simulink model "LGS_allFaultStuffDeleted"  (R2019b)
settings: Solver=FixedStepDiscrete  StartTime=0.0  StopTime=45.0  FixedStep=0.1  RelTol=1e-3
model workspace (MAT data in the model file):
  fipData : object (value not decoded)
  fipName : object (value not decoded)
  stepSize = 0.1
libraries: commrandsrc3 x16, simulink x3, LibFailureCondition x1
(part 5 of 7)

== stateflow chart LGS_allFaultStuffDeleted/Digital Part/Computing module1/GenericMonitoring8/GenericMonitoring2 ==
  state SensorValid
    entry: anomaly = false;
  state Channel1Invalid
  state SensorInvalid
    entry: anomaly = true;
  note: If at t the three channels are considered as valid and are equal, then the
      | value considered by the control software is this common value.
  state Channel2Invalid
  note: If a channel has been eliminated previously, and if at t the two remaining
      | channels are not equal, then the sensor is definitely considered as invalid.
  state Channel3Invalid
  note: If at t one channel is different from the two others for the first time (i.e.,
      | the three channels were considered as valid up to t), then this channel is
      | considered as invalid and is definitely eliminated. Only the two remaining
      | channels are considered in the future. At time t, the value considered by the
      | control software is the common value of the two remaining channels.
  (default) -> SensorValid
  SensorValid -> Channel1Invalid [order 1] : [(((Channel3&&Channel2) || ((~Channel3)&&(~Channel2))) && ((Channel1 && (~Channel2)) || ((~Channel1) && Channel2)))]
  Channel1Invalid -> SensorInvalid : [((Channel2 && (~Channel3)) || ((~Channel2) && Channel3))]
  SensorValid -> Channel2Invalid [order 2] : [(((Channel1&&Channel3) || ((~Channel1)&&(~Channel3))) && ((Channel1 && (~Channel2)) || ((~Channel1) && Channel2)))]
  SensorValid -> Channel3Invalid [order 3] : [(((Channel1&&Channel2) || ((~Channel1)&&(~Channel2))) && ((Channel1 && (~Channel3)) || ((~Channel1) && Channel3)))]
  Channel2Invalid -> SensorInvalid : [((Channel1 && (~Channel3)) || ((~Channel1) && Channel3))]
  Channel3Invalid -> SensorInvalid : [((Channel2 && (~Channel1)) || ((~Channel2) && Channel1))]
  data: Channel1 input boolean; Channel2 input boolean; Channel3 input boolean; anomaly output boolean

== stateflow chart LGS_allFaultStuffDeleted/Digital Part/Computing module1/GenericMonitoring9/GenericMonitoring2 ==
  state SensorValid
    entry: anomaly = false;
  state Channel1Invalid
  state SensorInvalid
    entry: anomaly = true;
  note: If at t the three channels are considered as valid and are equal, then the
      | value considered by the control software is this common value.
  state Channel2Invalid
  note: If a channel has been eliminated previously, and if at t the two remaining
      | channels are not equal, then the sensor is definitely considered as invalid.
  state Channel3Invalid
  note: If at t one channel is different from the two others for the first time (i.e.,
      | the three channels were considered as valid up to t), then this channel is
      | considered as invalid and is definitely eliminated. Only the two remaining
      | channels are considered in the future. At time t, the value considered by the
      | control software is the common value of the two remaining channels.
  (default) -> SensorValid
  SensorValid -> Channel1Invalid [order 1] : [(((Channel3&&Channel2) || ((~Channel3)&&(~Channel2))) && ((Channel1 && (~Channel2)) || ((~Channel1) && Channel2)))]
  Channel1Invalid -> SensorInvalid : [((Channel2 && (~Channel3)) || ((~Channel2) && Channel3))]
  SensorValid -> Channel2Invalid [order 2] : [(((Channel1&&Channel3) || ((~Channel1)&&(~Channel3))) && ((Channel1 && (~Channel2)) || ((~Channel1) && Channel2)))]
  SensorValid -> Channel3Invalid [order 3] : [(((Channel1&&Channel2) || ((~Channel1)&&(~Channel2))) && ((Channel1 && (~Channel3)) || ((~Channel1) && Channel3)))]
  Channel2Invalid -> SensorInvalid : [((Channel1 && (~Channel3)) || ((~Channel1) && Channel3))]
  Channel3Invalid -> SensorInvalid : [((Channel2 && (~Channel1)) || ((~Channel2) && Channel1))]
  data: Channel1 input boolean; Channel2 input boolean; Channel3 input boolean; anomaly output boolean

== stateflow chart LGS_allFaultStuffDeleted/Digital Part/Computing module1/GenericMonitoring15/GenericMonitoring2 ==
  state SensorValid
    entry: anomaly = false;
  state Channel1Invalid
  state SensorInvalid
    entry: anomaly = true;
  note: If at t the three channels are considered as valid and are equal, then the
      | value considered by the control software is this common value.
  state Channel2Invalid
  note: If a channel has been eliminated previously, and if at t the two remaining
      | channels are not equal, then the sensor is definitely considered as invalid.
  state Channel3Invalid
  note: If at t one channel is different from the two others for the first time (i.e.,
      | the three channels were considered as valid up to t), then this channel is
      | considered as invalid and is definitely eliminated. Only the two remaining
      | channels are considered in the future. At time t, the value considered by the
      | control software is the common value of the two remaining channels.
  (default) -> SensorValid
  SensorValid -> Channel1Invalid [order 1] : [(((Channel3&&Channel2) || ((~Channel3)&&(~Channel2))) && ((Channel1 && (~Channel2)) || ((~Channel1) && Channel2)))]
  Channel1Invalid -> SensorInvalid : [((Channel2 && (~Channel3)) || ((~Channel2) && Channel3))]
  SensorValid -> Channel2Invalid [order 2] : [(((Channel1&&Channel3) || ((~Channel1)&&(~Channel3))) && ((Channel1 && (~Channel2)) || ((~Channel1) && Channel2)))]
  SensorValid -> Channel3Invalid [order 3] : [(((Channel1&&Channel2) || ((~Channel1)&&(~Channel2))) && ((Channel1 && (~Channel3)) || ((~Channel1) && Channel3)))]
  Channel2Invalid -> SensorInvalid : [((Channel1 && (~Channel3)) || ((~Channel1) && Channel3))]
  Channel3Invalid -> SensorInvalid : [((Channel2 && (~Channel1)) || ((~Channel2) && Channel1))]
  data: Channel1 input boolean; Channel2 input boolean; Channel3 input boolean; anomaly output boolean

== stateflow chart LGS_allFaultStuffDeleted/Digital Part/Computing module1/GenericMonitoring16/GenericMonitoring2 ==
  state SensorValid
    entry: anomaly = false;
  state Channel1Invalid
  state SensorInvalid
    entry: anomaly = true;
  note: If at t the three channels are considered as valid and are equal, then the
      | value considered by the control software is this common value.
  state Channel2Invalid
  note: If a channel has been eliminated previously, and if at t the two remaining
      | channels are not equal, then the sensor is definitely considered as invalid.
  state Channel3Invalid
  note: If at t one channel is different from the two others for the first time (i.e.,
      | the three channels were considered as valid up to t), then this channel is
      | considered as invalid and is definitely eliminated. Only the two remaining
      | channels are considered in the future. At time t, the value considered by the
      | control software is the common value of the two remaining channels.
  (default) -> SensorValid
  SensorValid -> Channel1Invalid [order 1] : [(((Channel3&&Channel2) || ((~Channel3)&&(~Channel2))) && ((Channel1 && (~Channel2)) || ((~Channel1) && Channel2)))]
  Channel1Invalid -> SensorInvalid : [((Channel2 && (~Channel3)) || ((~Channel2) && Channel3))]
  SensorValid -> Channel2Invalid [order 2] : [(((Channel1&&Channel3) || ((~Channel1)&&(~Channel3))) && ((Channel1 && (~Channel2)) || ((~Channel1) && Channel2)))]
  SensorValid -> Channel3Invalid [order 3] : [(((Channel1&&Channel2) || ((~Channel1)&&(~Channel2))) && ((Channel1 && (~Channel3)) || ((~Channel1) && Channel3)))]
  Channel2Invalid -> SensorInvalid : [((Channel1 && (~Channel3)) || ((~Channel1) && Channel3))]
  Channel3Invalid -> SensorInvalid : [((Channel2 && (~Channel1)) || ((~Channel2) && Channel1))]
  data: Channel1 input boolean; Channel2 input boolean; Channel3 input boolean; anomaly output boolean

== stateflow chart LGS_allFaultStuffDeleted/Digital Part/Computing module2/AnalogicalSwitchMonitoring ==
  state SwitchOpened
    entry: time = int8(21);
    during: time = time -1;
  note: If the analogical switch is seen closed 1.5 second after a time interval of 20
      | seconds during which the handle position has not changed, then the switch
      | is considered as invalid.
  state Idle
    entry: anomaly = false;
  state HandleMoved
  state CounterOrder
  note: If the analogical switch is seen open 1 second after the handle position has
      | changed, then the switch is considered as invalid.
  state Anomaly
    entry: anomaly = true;
  (default) -> Idle
  SwitchOpened -> Idle [order 2] : [((time == 0) && (~SwitchSignal))]
  HandleMoved -> SwitchOpened [order 2] : [((SwitchSignal) && (~HandleMoved))]
  SwitchOpened -> CounterOrder [order 3] : [(HandleMoved)]
  SwitchOpened -> Anomaly [order 1] : [((time == 0) && (SwitchSignal))]
  Idle -> HandleMoved : [(HandleMoved)]
  HandleMoved -> CounterOrder [order 3] : [(HandleMoved)]
  CounterOrder -> HandleMoved
  HandleMoved -> Anomaly [order 1] : [((~SwitchSignal) && (~HandleMoved))]
  data: HandleMoved input boolean; time local int8 [0..21]; SwitchSignal input boolean; anomaly output boolean

== stateflow chart LGS_allFaultStuffDeleted/Digital Part/Computing module1/GenericMonitoring17/GenericMonitoring2 ==
  state SensorValid
    entry: anomaly = false;
  state Channel1Invalid
  state SensorInvalid
    entry: anomaly = true;
  note: If at t the three channels are considered as valid and are equal, then the
      | value considered by the control software is this common value.
  state Channel2Invalid
  note: If a channel has been eliminated previously, and if at t the two remaining
      | channels are not equal, then the sensor is definitely considered as invalid.
  state Channel3Invalid
  note: If at t one channel is different from the two others for the first time (i.e.,
      | the three channels were considered as valid up to t), then this channel is
      | considered as invalid and is definitely eliminated. Only the two remaining
      | channels are considered in the future. At time t, the value considered by the
      | control software is the common value of the two remaining channels.
  (default) -> SensorValid
  SensorValid -> Channel1Invalid [order 1] : [(((Channel3&&Channel2) || ((~Channel3)&&(~Channel2))) && ((Channel1 && (~Channel2)) || ((~Channel1) && Channel2)))]
  Channel1Invalid -> SensorInvalid : [((Channel2 && (~Channel3)) || ((~Channel2) && Channel3))]
  SensorValid -> Channel2Invalid [order 2] : [(((Channel1&&Channel3) || ((~Channel1)&&(~Channel3))) && ((Channel1 && (~Channel2)) || ((~Channel1) && Channel2)))]
  SensorValid -> Channel3Invalid [order 3] : [(((Channel1&&Channel2) || ((~Channel1)&&(~Channel2))) && ((Channel1 && (~Channel3)) || ((~Channel1) && Channel3)))]
  Channel2Invalid -> SensorInvalid : [((Channel1 && (~Channel3)) || ((~Channel1) && Channel3))]
  Channel3Invalid -> SensorInvalid : [((Channel2 && (~Channel1)) || ((~Channel2) && Channel1))]
  data: Channel1 input boolean; Channel2 input boolean; Channel3 input boolean; anomaly output boolean

== stateflow chart LGS_allFaultStuffDeleted/Digital Part/Computing module2/DoorMotionMonitoring ==
  state Idle
    entry: anomaly = false;
  state CloseDoors
    entry: time = int8(6);
    during: time = time -1;
  note: if the control software does not see the value door closed[x] = true for all
      | x ∈ {front, left, right} 7 seconds after stimulation of the closure electro-valve,
      | then the doors are considered as blocked and an anomaly is detected.
  state Succeeded
  state OpenDoors
    entry: time = int8(6);
    during: time = time - 1;
  note: if the control software does not see the value door open[x] = false for all x ∈ {front, left, right} 7 seconds after stimulation of the closure electro-valve, then the doors are considered as blocked and an anomaly is detected.
  state CounterOrder
  note: if the control software does not see the value door open[x] = true for all
      | x ∈ {front, left, right} 7 seconds after stimulation of the opening electrovalve,
      | then the doors are considered as blocked and an anomaly is detected.
  state DoorsBlocked
    entry: anomaly = true;
  note: if the control software does not see the value door closed[x] = false for all
      | x ∈ {front, left, right} 7 seconds after stimulation of the opening electro-valve,
      | then the doors are considered as blocked and an anomaly is detected.
  (default) -> Idle
  CloseDoors -> DoorsBlocked [order 2] : [((time == 0) && (~AllDoorsClosed))]
  Idle -> CloseDoors [order 2] : [((CloseDoorValve) && (~AllDoorsClosed))]
  CloseDoors -> DoorsBlocked [order 3] : [((time == 0) && (AllDoorsOpen))]
  Succeeded -> Idle
  CloseDoors -> Succeeded [order 1] : [(((time == 0) && (AllDoorsClosed)) && (~AllDoorsOpen))]
  CounterOrder -> CloseDoors [order 2] : [(CloseDoorValve)]
  CloseDoors -> CounterOrder [order 4] : [(~CloseDoorValve)]
  Idle -> OpenDoors [order 1] : [((OpenDoorValve) && (~AllDoorsOpen))]
  OpenDoors -> Succeeded [order 2] : [(((time == 0) && (~AllDoorsClosed)) && (AllDoorsOpen))]
  CounterOrder -> OpenDoors [order 1] : [(OpenDoorValve)]
  OpenDoors -> CounterOrder [order 4] : [(~OpenDoorValve)]
  OpenDoors -> DoorsBlocked [order 1] : [((time == 0) && (AllDoorsClosed))]
  OpenDoors -> DoorsBlocked [order 3] : [((time == 0) && (~AllDoorsOpen))]
  data: OpenDoorValve input boolean; time local int8 [0..6]; CloseDoorValve input boolean; anomaly output boolean; AllDoorsClosed input boolean; AllDoorsOpen input boolean

== stateflow chart LGS_allFaultStuffDeleted/Digital Part/Computing module2/GearMotionMonitoring ==
  state ContinueExtending
    entry: time = int8(2);
    during: time = time -1;
  note: if the control software does not see the value gear extended[x] = true for all x ∈ {front, left, right} 10 seconds after stimulation of the extension electrovalve, then the gears are considered as blocked and an anomaly is detected.
  state Idle
    entry: anomaly = false;
  state ExtendGears
    entry: time = int8(6);
    during: time = time -1;
  state RetractGears
    entry: time = int8(6);
    during: time = time - 1;
  state ContinueRetracting
    entry: time = int8(2);
    during: time = time -1;
  state Succeeded
  note: if the control software does not see the value gear retracted[x] = false for all x ∈ {front, left, right} 7 seconds after stimulation of the extension electrovalve, then the gears are considered as blocked and an anomaly is detected.
  state GearsBlocked
    entry: anomaly = true;
  state CounterOrder
  note: if the control software does not see the value gear retracted[x] = true for all x ∈ {front, left, right} 10 seconds after stimulation of the retraction electrovalve, then the gears are considered as blocked and an anomaly is detected.
  note: if the control software does not see the value gear extended[x] = false for all
      | x ∈ {front, left, right} 7 seconds after stimulation of the retraction electrovalve,
      | then the gears are considered as blocked and an anomaly is detected.
  (default) -> Idle
  ExtendGears -> ContinueExtending [order 1] : [((time == 0) && (~AllGearsRetracted))]
  Idle -> ExtendGears [order 2] : [(ExtensionValve)]
  ExtendGears -> GearsBlocked [order 2] : [((time == 0) && (AllGearsRetracted))]
  Succeeded -> Idle
  ExtendGears -> CounterOrder [order 3] : [(~ExtensionValve)]
  ContinueExtending -> GearsBlocked [order 2] : [((time == 0) && (~AllGearsExtended))]
  CounterOrder -> ExtendGears [order 2] : [(ExtensionValve)]
  Idle -> RetractGears [order 1] : [(RetractionValve)]
  ContinueExtending -> CounterOrder [order 3] : [(~ExtensionValve)]
  ContinueExtending -> Succeeded [order 1] : [((time == 0) && (AllGearsExtended))]
  RetractGears -> ContinueRetracting [order 2] : [((time == 0) && (~AllGearsExtended))]
  ContinueRetracting -> Succeeded [order 1] : [((time == 0) && (AllGearsRetracted))]
  CounterOrder -> RetractGears [order 1] : [(RetractionValve)]
  ContinueRetracting -> GearsBlocked [order 2] : [((time == 0) && (~AllGearsRetracted))]
  RetractGears -> GearsBlocked [order 1] : [((time == 0) && (AllGearsExtended))]
  RetractGears -> CounterOrder [order 3] : [(~RetractionValve)]
  ContinueRetracting -> CounterOrder [order 3] : [(~RetractionValve)]
  data: time local int8 [0..6]; anomaly output boolean; AllGearsExtended input boolean; AllGearsRetracted input boolean; ExtensionValve input boolean; RetractionValve input boolean

== stateflow chart LGS_allFaultStuffDeleted/Digital Part/Computing module2/GenericMonitoring/GenericMonitoring2 ==
  state SensorValid
    entry: anomaly = false;
  state Channel1Invalid
  state SensorInvalid
    entry: anomaly = true;
  note: If at t the three channels are considered as valid and are equal, then the
      | value considered by the control software is this common value.
  state Channel2Invalid
  note: If a channel has been eliminated previously, and if at t the two remaining
      | channels are not equal, then the sensor is definitely considered as invalid.
  state Channel3Invalid
  note: If at t one channel is different from the two others for the first time (i.e.,
      | the three channels were considered as valid up to t), then this channel is
      | considered as invalid and is definitely eliminated. Only the two remaining
      | channels are considered in the future. At time t, the value considered by the
      | control software is the common value of the two remaining channels.
  (default) -> SensorValid
  SensorValid -> Channel1Invalid [order 1] : [(((Channel3&&Channel2) || ((~Channel3)&&(~Channel2))) && ((Channel1 && (~Channel2)) || ((~Channel1) && Channel2)))]
  Channel1Invalid -> SensorInvalid : [((Channel2 && (~Channel3)) || ((~Channel2) && Channel3))]
  SensorValid -> Channel2Invalid [order 2] : [(((Channel1&&Channel3) || ((~Channel1)&&(~Channel3))) && ((Channel1 && (~Channel2)) || ((~Channel1) && Channel2)))]
  SensorValid -> Channel3Invalid [order 3] : [(((Channel1&&Channel2) || ((~Channel1)&&(~Channel2))) && ((Channel1 && (~Channel3)) || ((~Channel1) && Channel3)))]
  Channel2Invalid -> SensorInvalid : [((Channel1 && (~Channel3)) || ((~Channel1) && Channel3))]
  Channel3Invalid -> SensorInvalid : [((Channel2 && (~Channel1)) || ((~Channel2) && Channel1))]
  data: Channel1 input boolean; Channel2 input boolean; Channel3 input boolean; anomaly output boolean

== stateflow chart LGS_allFaultStuffDeleted/Digital Part/Computing module2/GenericMonitoring1/GenericMonitoring2 ==
  state SensorValid
    entry: anomaly = false;
  state Channel1Invalid
  state SensorInvalid
    entry: anomaly = true;
  note: If at t the three channels are considered as valid and are equal, then the
      | value considered by the control software is this common value.
  state Channel2Invalid
  note: If a channel has been eliminated previously, and if at t the two remaining
      | channels are not equal, then the sensor is definitely considered as invalid.
  state Channel3Invalid
  note: If at t one channel is different from the two others for the first time (i.e.,
      | the three channels were considered as valid up to t), then this channel is
      | considered as invalid and is definitely eliminated. Only the two remaining
      | channels are considered in the future. At time t, the value considered by the
      | control software is the common value of the two remaining channels.
  (default) -> SensorValid
  SensorValid -> Channel1Invalid [order 1] : [(((Channel3&&Channel2) || ((~Channel3)&&(~Channel2))) && ((Channel1 && (~Channel2)) || ((~Channel1) && Channel2)))]
  Channel1Invalid -> SensorInvalid : [((Channel2 && (~Channel3)) || ((~Channel2) && Channel3))]
  SensorValid -> Channel2Invalid [order 2] : [(((Channel1&&Channel3) || ((~Channel1)&&(~Channel3))) && ((Channel1 && (~Channel2)) || ((~Channel1) && Channel2)))]
  SensorValid -> Channel3Invalid [order 3] : [(((Channel1&&Channel2) || ((~Channel1)&&(~Channel2))) && ((Channel1 && (~Channel3)) || ((~Channel1) && Channel3)))]
  Channel2Invalid -> SensorInvalid : [((Channel1 && (~Channel3)) || ((~Channel1) && Channel3))]
  Channel3Invalid -> SensorInvalid : [((Channel2 && (~Channel1)) || ((~Channel2) && Channel1))]
  data: Channel1 input boolean; Channel2 input boolean; Channel3 input boolean; anomaly output boolean

== stateflow chart LGS_allFaultStuffDeleted/Digital Part/Computing module2/GenericMonitoring10/GenericMonitoring2 ==
  state SensorValid
    entry: anomaly = false;
  state Channel1Invalid
  state SensorInvalid
    entry: anomaly = true;
  note: If at t the three channels are considered as valid and are equal, then the
      | value considered by the control software is this common value.
  state Channel2Invalid
  note: If a channel has been eliminated previously, and if at t the two remaining
      | channels are not equal, then the sensor is definitely considered as invalid.
  state Channel3Invalid
  note: If at t one channel is different from the two others for the first time (i.e.,
      | the three channels were considered as valid up to t), then this channel is
      | considered as invalid and is definitely eliminated. Only the two remaining
      | channels are considered in the future. At time t, the value considered by the
      | control software is the common value of the two remaining channels.
  (default) -> SensorValid
  SensorValid -> Channel1Invalid [order 1] : [(((Channel3&&Channel2) || ((~Channel3)&&(~Channel2))) && ((Channel1 && (~Channel2)) || ((~Channel1) && Channel2)))]
  Channel1Invalid -> SensorInvalid : [((Channel2 && (~Channel3)) || ((~Channel2) && Channel3))]
  SensorValid -> Channel2Invalid [order 2] : [(((Channel1&&Channel3) || ((~Channel1)&&(~Channel3))) && ((Channel1 && (~Channel2)) || ((~Channel1) && Channel2)))]
  SensorValid -> Channel3Invalid [order 3] : [(((Channel1&&Channel2) || ((~Channel1)&&(~Channel2))) && ((Channel1 && (~Channel3)) || ((~Channel1) && Channel3)))]
  Channel2Invalid -> SensorInvalid : [((Channel1 && (~Channel3)) || ((~Channel1) && Channel3))]
  Channel3Invalid -> SensorInvalid : [((Channel2 && (~Channel1)) || ((~Channel2) && Channel1))]
  data: Channel1 input boolean; Channel2 input boolean; Channel3 input boolean; anomaly output boolean

== stateflow chart LGS_allFaultStuffDeleted/Digital Part/Computing module2/GenericMonitoring11/GenericMonitoring2 ==
  state SensorValid
    entry: anomaly = false;
  state Channel1Invalid
  state SensorInvalid
    entry: anomaly = true;
  note: If at t the three channels are considered as valid and are equal, then the
      | value considered by the control software is this common value.
  state Channel2Invalid
  note: If a channel has been eliminated previously, and if at t the two remaining
      | channels are not equal, then the sensor is definitely considered as invalid.
  state Channel3Invalid
  note: If at t one channel is different from the two others for the first time (i.e.,
      | the three channels were considered as valid up to t), then this channel is
      | considered as invalid and is definitely eliminated. Only the two remaining
      | channels are considered in the future. At time t, the value considered by the
      | control software is the common value of the two remaining channels.
  (default) -> SensorValid
  SensorValid -> Channel1Invalid [order 1] : [(((Channel3&&Channel2) || ((~Channel3)&&(~Channel2))) && ((Channel1 && (~Channel2)) || ((~Channel1) && Channel2)))]
  Channel1Invalid -> SensorInvalid : [((Channel2 && (~Channel3)) || ((~Channel2) && Channel3))]
  SensorValid -> Channel2Invalid [order 2] : [(((Channel1&&Channel3) || ((~Channel1)&&(~Channel3))) && ((Channel1 && (~Channel2)) || ((~Channel1) && Channel2)))]
  SensorValid -> Channel3Invalid [order 3] : [(((Channel1&&Channel2) || ((~Channel1)&&(~Channel2))) && ((Channel1 && (~Channel3)) || ((~Channel1) && Channel3)))]
  Channel2Invalid -> SensorInvalid : [((Channel1 && (~Channel3)) || ((~Channel1) && Channel3))]
  Channel3Invalid -> SensorInvalid : [((Channel2 && (~Channel1)) || ((~Channel2) && Channel1))]
  data: Channel1 input boolean; Channel2 input boolean; Channel3 input boolean; anomaly output boolean

== stateflow chart LGS_allFaultStuffDeleted/Digital Part/Computing module2/GenericMonitoring12/GenericMonitoring2 ==
  state SensorValid
    entry: anomaly = false;
  state Channel1Invalid
  state SensorInvalid
    entry: anomaly = true;
  note: If at t the three channels are considered as valid and are equal, then the
      | value considered by the control software is this common value.
  state Channel2Invalid
  note: If a channel has been eliminated previously, and if at t the two remaining
      | channels are not equal, then the sensor is definitely considered as invalid.
  state Channel3Invalid
  note: If at t one channel is different from the two others for the first time (i.e.,
      | the three channels were considered as valid up to t), then this channel is
      | considered as invalid and is definitely eliminated. Only the two remaining
      | channels are considered in the future. At time t, the value considered by the
      | control software is the common value of the two remaining channels.
  (default) -> SensorValid
  SensorValid -> Channel1Invalid [order 1] : [(((Channel3&&Channel2) || ((~Channel3)&&(~Channel2))) && ((Channel1 && (~Channel2)) || ((~Channel1) && Channel2)))]
  Channel1Invalid -> SensorInvalid : [((Channel2 && (~Channel3)) || ((~Channel2) && Channel3))]
  SensorValid -> Channel2Invalid [order 2] : [(((Channel1&&Channel3) || ((~Channel1)&&(~Channel3))) && ((Channel1 && (~Channel2)) || ((~Channel1) && Channel2)))]
  SensorValid -> Channel3Invalid [order 3] : [(((Channel1&&Channel2) || ((~Channel1)&&(~Channel2))) && ((Channel1 && (~Channel3)) || ((~Channel1) && Channel3)))]
  Channel2Invalid -> SensorInvalid : [((Channel1 && (~Channel3)) || ((~Channel1) && Channel3))]
  Channel3Invalid -> SensorInvalid : [((Channel2 && (~Channel1)) || ((~Channel2) && Channel1))]
  data: Channel1 input boolean; Channel2 input boolean; Channel3 input boolean; anomaly output boolean

== stateflow chart LGS_allFaultStuffDeleted/Digital Part/Computing module2/GenericMonitoring13/GenericMonitoring2 ==
  state SensorValid
    entry: anomaly = false;
  state Channel1Invalid
  state SensorInvalid
    entry: anomaly = true;
  note: If at t the three channels are considered as valid and are equal, then the
      | value considered by the control software is this common value.
  state Channel2Invalid
  note: If a channel has been eliminated previously, and if at t the two remaining
      | channels are not equal, then the sensor is definitely considered as invalid.
  state Channel3Invalid
  note: If at t one channel is different from the two others for the first time (i.e.,
      | the three channels were considered as valid up to t), then this channel is
      | considered as invalid and is definitely eliminated. Only the two remaining
      | channels are considered in the future. At time t, the value considered by the
      | control software is the common value of the two remaining channels.
  (default) -> SensorValid
  SensorValid -> Channel1Invalid [order 1] : [(((Channel3&&Channel2) || ((~Channel3)&&(~Channel2))) && ((Channel1 && (~Channel2)) || ((~Channel1) && Channel2)))]
  Channel1Invalid -> SensorInvalid : [((Channel2 && (~Channel3)) || ((~Channel2) && Channel3))]
  SensorValid -> Channel2Invalid [order 2] : [(((Channel1&&Channel3) || ((~Channel1)&&(~Channel3))) && ((Channel1 && (~Channel2)) || ((~Channel1) && Channel2)))]
  SensorValid -> Channel3Invalid [order 3] : [(((Channel1&&Channel2) || ((~Channel1)&&(~Channel2))) && ((Channel1 && (~Channel3)) || ((~Channel1) && Channel3)))]
  Channel2Invalid -> SensorInvalid : [((Channel1 && (~Channel3)) || ((~Channel1) && Channel3))]
  Channel3Invalid -> SensorInvalid : [((Channel2 && (~Channel1)) || ((~Channel2) && Channel1))]
  data: Channel1 input boolean; Channel2 input boolean; Channel3 input boolean; anomaly output boolean

== stateflow chart LGS_allFaultStuffDeleted/Digital Part/Computing module2/GenericMonitoring14/GenericMonitoring2 ==
  state SensorValid
    entry: anomaly = false;
  state Channel1Invalid
  state SensorInvalid
    entry: anomaly = true;
  note: If at t the three channels are considered as valid and are equal, then the
      | value considered by the control software is this common value.
  state Channel2Invalid
  note: If a channel has been eliminated previously, and if at t the two remaining
      | channels are not equal, then the sensor is definitely considered as invalid.
  state Channel3Invalid
  note: If at t one channel is different from the two others for the first time (i.e.,
      | the three channels were considered as valid up to t), then this channel is
      | considered as invalid and is definitely eliminated. Only the two remaining
      | channels are considered in the future. At time t, the value considered by the
      | control software is the common value of the two remaining channels.
  (default) -> SensorValid
  SensorValid -> Channel1Invalid [order 1] : [(((Channel3&&Channel2) || ((~Channel3)&&(~Channel2))) && ((Channel1 && (~Channel2)) || ((~Channel1) && Channel2)))]
  Channel1Invalid -> SensorInvalid : [((Channel2 && (~Channel3)) || ((~Channel2) && Channel3))]
  SensorValid -> Channel2Invalid [order 2] : [(((Channel1&&Channel3) || ((~Channel1)&&(~Channel3))) && ((Channel1 && (~Channel2)) || ((~Channel1) && Channel2)))]
  SensorValid -> Channel3Invalid [order 3] : [(((Channel1&&Channel2) || ((~Channel1)&&(~Channel2))) && ((Channel1 && (~Channel3)) || ((~Channel1) && Channel3)))]
  Channel2Invalid -> SensorInvalid : [((Channel1 && (~Channel3)) || ((~Channel1) && Channel3))]
  Channel3Invalid -> SensorInvalid : [((Channel2 && (~Channel1)) || ((~Channel2) && Channel1))]
  data: Channel1 input boolean; Channel2 input boolean; Channel3 input boolean; anomaly output boolean

== stateflow chart LGS_allFaultStuffDeleted/Digital Part/Computing module2/GenericMonitoring15/GenericMonitoring2 ==
  state SensorValid
    entry: anomaly = false;
  state Channel1Invalid
  state SensorInvalid
    entry: anomaly = true;
  note: If at t the three channels are considered as valid and are equal, then the
      | value considered by the control software is this common value.
  state Channel2Invalid
  note: If a channel has been eliminated previously, and if at t the two remaining
      | channels are not equal, then the sensor is definitely considered as invalid.
  state Channel3Invalid
  note: If at t one channel is different from the two others for the first time (i.e.,
      | the three channels were considered as valid up to t), then this channel is
      | considered as invalid and is definitely eliminated. Only the two remaining
      | channels are considered in the future. At time t, the value considered by the
      | control software is the common value of the two remaining channels.
  (default) -> SensorValid
  SensorValid -> Channel1Invalid [order 1] : [(((Channel3&&Channel2) || ((~Channel3)&&(~Channel2))) && ((Channel1 && (~Channel2)) || ((~Channel1) && Channel2)))]
  Channel1Invalid -> SensorInvalid : [((Channel2 && (~Channel3)) || ((~Channel2) && Channel3))]
  SensorValid -> Channel2Invalid [order 2] : [(((Channel1&&Channel3) || ((~Channel1)&&(~Channel3))) && ((Channel1 && (~Channel2)) || ((~Channel1) && Channel2)))]
  SensorValid -> Channel3Invalid [order 3] : [(((Channel1&&Channel2) || ((~Channel1)&&(~Channel2))) && ((Channel1 && (~Channel3)) || ((~Channel1) && Channel3)))]
  Channel2Invalid -> SensorInvalid : [((Channel1 && (~Channel3)) || ((~Channel1) && Channel3))]
  Channel3Invalid -> SensorInvalid : [((Channel2 && (~Channel1)) || ((~Channel2) && Channel1))]
  data: Channel1 input boolean; Channel2 input boolean; Channel3 input boolean; anomaly output boolean

== stateflow chart LGS_allFaultStuffDeleted/Digital Part/Computing module2/GenericMonitoring16/GenericMonitoring2 ==
  state SensorValid
    entry: anomaly = false;
  state Channel1Invalid
  state SensorInvalid
    entry: anomaly = true;
  note: If at t the three channels are considered as valid and are equal, then the
      | value considered by the control software is this common value.
  state Channel2Invalid
  note: If a channel has been eliminated previously, and if at t the two remaining
      | channels are not equal, then the sensor is definitely considered as invalid.
  state Channel3Invalid
  note: If at t one channel is different from the two others for the first time (i.e.,
      | the three channels were considered as valid up to t), then this channel is
      | considered as invalid and is definitely eliminated. Only the two remaining
      | channels are considered in the future. At time t, the value considered by the
      | control software is the common value of the two remaining channels.
  (default) -> SensorValid
  SensorValid -> Channel1Invalid [order 1] : [(((Channel3&&Channel2) || ((~Channel3)&&(~Channel2))) && ((Channel1 && (~Channel2)) || ((~Channel1) && Channel2)))]
  Channel1Invalid -> SensorInvalid : [((Channel2 && (~Channel3)) || ((~Channel2) && Channel3))]
  SensorValid -> Channel2Invalid [order 2] : [(((Channel1&&Channel3) || ((~Channel1)&&(~Channel3))) && ((Channel1 && (~Channel2)) || ((~Channel1) && Channel2)))]
  SensorValid -> Channel3Invalid [order 3] : [(((Channel1&&Channel2) || ((~Channel1)&&(~Channel2))) && ((Channel1 && (~Channel3)) || ((~Channel1) && Channel3)))]
  Channel2Invalid -> SensorInvalid : [((Channel1 && (~Channel3)) || ((~Channel1) && Channel3))]
  Channel3Invalid -> SensorInvalid : [((Channel2 && (~Channel1)) || ((~Channel2) && Channel1))]
  data: Channel1 input boolean; Channel2 input boolean; Channel3 input boolean; anomaly output boolean

== stateflow chart LGS_allFaultStuffDeleted/Digital Part/Computing module2/GenericMonitoring17/GenericMonitoring2 ==
  state SensorValid
    entry: anomaly = false;
  state Channel1Invalid
  state SensorInvalid
    entry: anomaly = true;
  note: If at t the three channels are considered as valid and are equal, then the
      | value considered by the control software is this common value.
  state Channel2Invalid
  note: If a channel has been eliminated previously, and if at t the two remaining
      | channels are not equal, then the sensor is definitely considered as invalid.
  state Channel3Invalid
  note: If at t one channel is different from the two others for the first time (i.e.,
      | the three channels were considered as valid up to t), then this channel is
      | considered as invalid and is definitely eliminated. Only the two remaining
      | channels are considered in the future. At time t, the value considered by the
      | control software is the common value of the two remaining channels.
  (default) -> SensorValid
  SensorValid -> Channel1Invalid [order 1] : [(((Channel3&&Channel2) || ((~Channel3)&&(~Channel2))) && ((Channel1 && (~Channel2)) || ((~Channel1) && Channel2)))]
  Channel1Invalid -> SensorInvalid : [((Channel2 && (~Channel3)) || ((~Channel2) && Channel3))]
  SensorValid -> Channel2Invalid [order 2] : [(((Channel1&&Channel3) || ((~Channel1)&&(~Channel3))) && ((Channel1 && (~Channel2)) || ((~Channel1) && Channel2)))]
  SensorValid -> Channel3Invalid [order 3] : [(((Channel1&&Channel2) || ((~Channel1)&&(~Channel2))) && ((Channel1 && (~Channel3)) || ((~Channel1) && Channel3)))]
  Channel2Invalid -> SensorInvalid : [((Channel1 && (~Channel3)) || ((~Channel1) && Channel3))]
  Channel3Invalid -> SensorInvalid : [((Channel2 && (~Channel1)) || ((~Channel2) && Channel1))]
  data: Channel1 input boolean; Channel2 input boolean; Channel3 input boolean; anomaly output boolean

== stateflow chart LGS_allFaultStuffDeleted/Digital Part/Computing module2/GenericMonitoring2/GenericMonitoring2 ==
  state SensorValid
    entry: anomaly = false;
  state Channel1Invalid
  state SensorInvalid
    entry: anomaly = true;
  note: If at t the three channels are considered as valid and are equal, then the
      | value considered by the control software is this common value.
  state Channel2Invalid
  note: If a channel has been eliminated previously, and if at t the two remaining
      | channels are not equal, then the sensor is definitely considered as invalid.
  state Channel3Invalid
  note: If at t one channel is different from the two others for the first time (i.e.,
      | the three channels were considered as valid up to t), then this channel is
      | considered as invalid and is definitely eliminated. Only the two remaining
      | channels are considered in the future. At time t, the value considered by the
      | control software is the common value of the two remaining channels.
  (default) -> SensorValid
  SensorValid -> Channel1Invalid [order 1] : [(((Channel3&&Channel2) || ((~Channel3)&&(~Channel2))) && ((Channel1 && (~Channel2)) || ((~Channel1) && Channel2)))]
  Channel1Invalid -> SensorInvalid : [((Channel2 && (~Channel3)) || ((~Channel2) && Channel3))]
  SensorValid -> Channel2Invalid [order 2] : [(((Channel1&&Channel3) || ((~Channel1)&&(~Channel3))) && ((Channel1 && (~Channel2)) || ((~Channel1) && Channel2)))]
  SensorValid -> Channel3Invalid [order 3] : [(((Channel1&&Channel2) || ((~Channel1)&&(~Channel2))) && ((Channel1 && (~Channel3)) || ((~Channel1) && Channel3)))]
  Channel2Invalid -> SensorInvalid : [((Channel1 && (~Channel3)) || ((~Channel1) && Channel3))]
  Channel3Invalid -> SensorInvalid : [((Channel2 && (~Channel1)) || ((~Channel2) && Channel1))]
  data: Channel1 input boolean; Channel2 input boolean; Channel3 input boolean; anomaly output boolean

== stateflow chart LGS_allFaultStuffDeleted/Digital Part/Computing module2/GenericMonitoring3/GenericMonitoring2 ==
  state SensorValid
    entry: anomaly = false;
  state Channel1Invalid
  state SensorInvalid
    entry: anomaly = true;
  note: If at t the three channels are considered as valid and are equal, then the
      | value considered by the control software is this common value.
  state Channel2Invalid
  note: If a channel has been eliminated previously, and if at t the two remaining
      | channels are not equal, then the sensor is definitely considered as invalid.
  state Channel3Invalid
  note: If at t one channel is different from the two others for the first time (i.e.,
      | the three channels were considered as valid up to t), then this channel is
      | considered as invalid and is definitely eliminated. Only the two remaining
      | channels are considered in the future. At time t, the value considered by the
      | control software is the common value of the two remaining channels.
  (default) -> SensorValid
  SensorValid -> Channel1Invalid [order 1] : [(((Channel3&&Channel2) || ((~Channel3)&&(~Channel2))) && ((Channel1 && (~Channel2)) || ((~Channel1) && Channel2)))]
  Channel1Invalid -> SensorInvalid : [((Channel2 && (~Channel3)) || ((~Channel2) && Channel3))]
  SensorValid -> Channel2Invalid [order 2] : [(((Channel1&&Channel3) || ((~Channel1)&&(~Channel3))) && ((Channel1 && (~Channel2)) || ((~Channel1) && Channel2)))]
  SensorValid -> Channel3Invalid [order 3] : [(((Channel1&&Channel2) || ((~Channel1)&&(~Channel2))) && ((Channel1 && (~Channel3)) || ((~Channel1) && Channel3)))]
  Channel2Invalid -> SensorInvalid : [((Channel1 && (~Channel3)) || ((~Channel1) && Channel3))]
  Channel3Invalid -> SensorInvalid : [((Channel2 && (~Channel1)) || ((~Channel2) && Channel1))]
  data: Channel1 input boolean; Channel2 input boolean; Channel3 input boolean; anomaly output boolean

== stateflow chart LGS_allFaultStuffDeleted/Digital Part/Computing module2/GenericMonitoring4/GenericMonitoring2 ==
  state SensorValid
    entry: anomaly = false;
  state Channel1Invalid
  state SensorInvalid
    entry: anomaly = true;
  note: If at t the three channels are considered as valid and are equal, then the
      | value considered by the control software is this common value.
  state Channel2Invalid
  note: If a channel has been eliminated previously, and if at t the two remaining
      | channels are not equal, then the sensor is definitely considered as invalid.
  state Channel3Invalid
  note: If at t one channel is different from the two others for the first time (i.e.,
      | the three channels were considered as valid up to t), then this channel is
      | considered as invalid and is definitely eliminated. Only the two remaining
      | channels are considered in the future. At time t, the value considered by the
      | control software is the common value of the two remaining channels.
  (default) -> SensorValid
  SensorValid -> Channel1Invalid [order 1] : [(((Channel3&&Channel2) || ((~Channel3)&&(~Channel2))) && ((Channel1 && (~Channel2)) || ((~Channel1) && Channel2)))]
  Channel1Invalid -> SensorInvalid : [((Channel2 && (~Channel3)) || ((~Channel2) && Channel3))]
  SensorValid -> Channel2Invalid [order 2] : [(((Channel1&&Channel3) || ((~Channel1)&&(~Channel3))) && ((Channel1 && (~Channel2)) || ((~Channel1) && Channel2)))]
  SensorValid -> Channel3Invalid [order 3] : [(((Channel1&&Channel2) || ((~Channel1)&&(~Channel2))) && ((Channel1 && (~Channel3)) || ((~Channel1) && Channel3)))]
  Channel2Invalid -> SensorInvalid : [((Channel1 && (~Channel3)) || ((~Channel1) && Channel3))]
  Channel3Invalid -> SensorInvalid : [((Channel2 && (~Channel1)) || ((~Channel2) && Channel1))]
  data: Channel1 input boolean; Channel2 input boolean; Channel3 input boolean; anomaly output boolean

== stateflow chart LGS_allFaultStuffDeleted/Digital Part/Computing module2/GenericMonitoring5/GenericMonitoring2 ==
  state SensorValid
    entry: anomaly = false;
  state Channel1Invalid
  state SensorInvalid
    entry: anomaly = true;
  note: If at t the three channels are considered as valid and are equal, then the
      | value considered by the control software is this common value.
  state Channel2Invalid
  note: If a channel has been eliminated previously, and if at t the two remaining
      | channels are not equal, then the sensor is definitely considered as invalid.
  state Channel3Invalid
  note: If at t one channel is different from the two others for the first time (i.e.,
      | the three channels were considered as valid up to t), then this channel is
      | considered as invalid and is definitely eliminated. Only the two remaining
      | channels are considered in the future. At time t, the value considered by the
      | control software is the common value of the two remaining channels.
  (default) -> SensorValid
  SensorValid -> Channel1Invalid [order 1] : [(((Channel3&&Channel2) || ((~Channel3)&&(~Channel2))) && ((Channel1 && (~Channel2)) || ((~Channel1) && Channel2)))]
  Channel1Invalid -> SensorInvalid : [((Channel2 && (~Channel3)) || ((~Channel2) && Channel3))]
  SensorValid -> Channel2Invalid [order 2] : [(((Channel1&&Channel3) || ((~Channel1)&&(~Channel3))) && ((Channel1 && (~Channel2)) || ((~Channel1) && Channel2)))]
  SensorValid -> Channel3Invalid [order 3] : [(((Channel1&&Channel2) || ((~Channel1)&&(~Channel2))) && ((Channel1 && (~Channel3)) || ((~Channel1) && Channel3)))]
  Channel2Invalid -> SensorInvalid : [((Channel1 && (~Channel3)) || ((~Channel1) && Channel3))]
  Channel3Invalid -> SensorInvalid : [((Channel2 && (~Channel1)) || ((~Channel2) && Channel1))]
  data: Channel1 input boolean; Channel2 input boolean; Channel3 input boolean; anomaly output boolean

== stateflow chart LGS_allFaultStuffDeleted/Digital Part/Computing module2/GenericMonitoring6/GenericMonitoring2 ==
  state SensorValid
    entry: anomaly = false;
  state Channel1Invalid
  state SensorInvalid
    entry: anomaly = true;
  note: If at t the three channels are considered as valid and are equal, then the
      | value considered by the control software is this common value.
  state Channel2Invalid
  note: If a channel has been eliminated previously, and if at t the two remaining
      | channels are not equal, then the sensor is definitely considered as invalid.
  state Channel3Invalid
  note: If at t one channel is different from the two others for the first time (i.e.,
      | the three channels were considered as valid up to t), then this channel is
      | considered as invalid and is definitely eliminated. Only the two remaining
      | channels are considered in the future. At time t, the value considered by the
      | control software is the common value of the two remaining channels.
  (default) -> SensorValid
  SensorValid -> Channel1Invalid [order 1] : [(((Channel3&&Channel2) || ((~Channel3)&&(~Channel2))) && ((Channel1 && (~Channel2)) || ((~Channel1) && Channel2)))]
  Channel1Invalid -> SensorInvalid : [((Channel2 && (~Channel3)) || ((~Channel2) && Channel3))]
  SensorValid -> Channel2Invalid [order 2] : [(((Channel1&&Channel3) || ((~Channel1)&&(~Channel3))) && ((Channel1 && (~Channel2)) || ((~Channel1) && Channel2)))]
  SensorValid -> Channel3Invalid [order 3] : [(((Channel1&&Channel2) || ((~Channel1)&&(~Channel2))) && ((Channel1 && (~Channel3)) || ((~Channel1) && Channel3)))]
  Channel2Invalid -> SensorInvalid : [((Channel1 && (~Channel3)) || ((~Channel1) && Channel3))]
  Channel3Invalid -> SensorInvalid : [((Channel2 && (~Channel1)) || ((~Channel2) && Channel1))]
  data: Channel1 input boolean; Channel2 input boolean; Channel3 input boolean; anomaly output boolean

== stateflow chart LGS_allFaultStuffDeleted/Digital Part/Computing module2/GenericMonitoring7/GenericMonitoring2 ==
  state SensorValid
    entry: anomaly = false;
  state Channel1Invalid
  state SensorInvalid
    entry: anomaly = true;
  note: If at t the three channels are considered as valid and are equal, then the
      | value considered by the control software is this common value.
  state Channel2Invalid
  note: If a channel has been eliminated previously, and if at t the two remaining
      | channels are not equal, then the sensor is definitely considered as invalid.
  state Channel3Invalid
  note: If at t one channel is different from the two others for the first time (i.e.,
      | the three channels were considered as valid up to t), then this channel is
      | considered as invalid and is definitely eliminated. Only the two remaining
      | channels are considered in the future. At time t, the value considered by the
      | control software is the common value of the two remaining channels.
  (default) -> SensorValid
  SensorValid -> Channel1Invalid [order 1] : [(((Channel3&&Channel2) || ((~Channel3)&&(~Channel2))) && ((Channel1 && (~Channel2)) || ((~Channel1) && Channel2)))]
  Channel1Invalid -> SensorInvalid : [((Channel2 && (~Channel3)) || ((~Channel2) && Channel3))]
  SensorValid -> Channel2Invalid [order 2] : [(((Channel1&&Channel3) || ((~Channel1)&&(~Channel3))) && ((Channel1 && (~Channel2)) || ((~Channel1) && Channel2)))]
  SensorValid -> Channel3Invalid [order 3] : [(((Channel1&&Channel2) || ((~Channel1)&&(~Channel2))) && ((Channel1 && (~Channel3)) || ((~Channel1) && Channel3)))]
  Channel2Invalid -> SensorInvalid : [((Channel1 && (~Channel3)) || ((~Channel1) && Channel3))]
  Channel3Invalid -> SensorInvalid : [((Channel2 && (~Channel1)) || ((~Channel2) && Channel1))]
  data: Channel1 input boolean; Channel2 input boolean; Channel3 input boolean; anomaly output boolean

== stateflow chart LGS_allFaultStuffDeleted/Digital Part/Computing module2/GenericMonitoring8/GenericMonitoring2 ==
  state SensorValid
    entry: anomaly = false;
  state Channel1Invalid
  state SensorInvalid
    entry: anomaly = true;
  note: If at t the three channels are considered as valid and are equal, then the
      | value considered by the control software is this common value.
  state Channel2Invalid
  note: If a channel has been eliminated previously, and if at t the two remaining
      | channels are not equal, then the sensor is definitely considered as invalid.
  state Channel3Invalid
  note: If at t one channel is different from the two others for the first time (i.e.,
      | the three channels were considered as valid up to t), then this channel is
      | considered as invalid and is definitely eliminated. Only the two remaining
      | channels are considered in the future. At time t, the value considered by the
      | control software is the common value of the two remaining channels.
  (default) -> SensorValid
  SensorValid -> Channel1Invalid [order 1] : [(((Channel3&&Channel2) || ((~Channel3)&&(~Channel2))) && ((Channel1 && (~Channel2)) || ((~Channel1) && Channel2)))]
  Channel1Invalid -> SensorInvalid : [((Channel2 && (~Channel3)) || ((~Channel2) && Channel3))]
  SensorValid -> Channel2Invalid [order 2] : [(((Channel1&&Channel3) || ((~Channel1)&&(~Channel3))) && ((Channel1 && (~Channel2)) || ((~Channel1) && Channel2)))]
  SensorValid -> Channel3Invalid [order 3] : [(((Channel1&&Channel2) || ((~Channel1)&&(~Channel2))) && ((Channel1 && (~Channel3)) || ((~Channel1) && Channel3)))]
  Channel2Invalid -> SensorInvalid : [((Channel1 && (~Channel3)) || ((~Channel1) && Channel3))]
  Channel3Invalid -> SensorInvalid : [((Channel2 && (~Channel1)) || ((~Channel2) && Channel1))]
  data: Channel1 input boolean; Channel2 input boolean; Channel3 input boolean; anomaly output boolean
